simulink model "Experiment_2_cs"  (Simulink 8.4)
settings: Solver=ode5  SolverMode=SingleTasking  StartTime=0.0  StopTime=inf  FixedStep=1/100  RelTol=1e-3
PreLoadFcn:
  | mbxruntime.callbacks.PreLoadFcn(bdroot);
PostLoadFcn:
  | mbxruntime.callbacks.PostLoadFcn(bdroot);
InitFcn:
  | mbxruntime.callbacks.InitFcn(bdroot);
StartFcn:
  | mbxruntime.callbacks.StartFcn(bdroot);
StopFcn:
  | mbxruntime.callbacks.StopFcn(bdroot);
undefined symbols (not defined in the file or in its folder): dfreq, gray, InitImageOutputDir, Rec, SDTV, strel, warningInitialVelocity, x0
libraries: simulink x43, PreScanSimulinkLibrary x19, visiontextngfix x15, simulink_extras x11, visionconversions x3, PreScanUsefulBlocks x3, visionsinks x2, visionstatistics x1, visionmorphops x1, visionanalysis x1
(part 8 of 8)

== matlab function Audi_A8_1/ENABLED/PPS Model/Pedestrian detection/Blob Analysis/PEDES1 ==
  data: inpoints output double; pts input double
function inpoints= points(pts)
%#eml
inpoints = pts;
inpoints(1, :)=pts(2, :);
inpoints(2, :)=pts(1, :);

for i = 1 : size(inpoints, 2)
    if inpoints(1, i) ~= -1
        inpoints(1, i)=inpoints(1, i) +1;
    end
    if inpoints(2, i) ~= -1
        inpoints(2, i)=inpoints(2, i) +1;
    end
end

== matlab function Audi_A8_1/ENABLED/V2X_210_Generic_Expander/Expander ==
  data: u input Bus: PRESCAN_V2X_USER_GENERIC_MESSAGE; y output Bus: PRESCAN_V2X_FIXED_GENERIC_MESSAGE; z input Bus: PRESCAN_V2X_FIXED_GENERIC_MESSAGE
function y = fcn(u, z)
%#eml

y = V2X_GENERIC_expander(u, z);

== matlab function Audi_A8_1/ENABLED/PathFollower_Preview_1/LateralController/Calculate delta steering error/eml_delta_steering_error ==
  data: v_x_vehicle input double; v_x_vehicle_Min input double; t_Preview_LatCtrl input double; delta_steeringwheeltotal output double; v_y_vehicle input double; yawrate_vehicle input double; CorneringStiffness_Tyres_Front input double; CorneringStiffness_Tyres_Rear input double; m_vehicle_total input double; inertia_z_vehicle_total input double; e_Lat input double size=10; Pos_x_CoG_Vehicle input double; wheelbase input double; RefreshCounter parameter double
function delta_steeringwheeltotal = eml_delta_steering_error(v_x_vehicle,v_x_vehicle_Min,t_Preview_LatCtrl,v_y_vehicle,yawrate_vehicle,CorneringStiffness_Tyres_Front,CorneringStiffness_Tyres_Rear,m_vehicle_total,inertia_z_vehicle_total,e_Lat,Pos_x_CoG_Vehicle,wheelbase,RefreshCounter)

delta_steeringwheeltotal = emlfcn_delta_steering_error(v_x_vehicle,v_x_vehicle_Min,t_Preview_LatCtrl,v_y_vehicle,yawrate_vehicle,CorneringStiffness_Tyres_Front,CorneringStiffness_Tyres_Rear,m_vehicle_total,inertia_z_vehicle_total,e_Lat,Pos_x_CoG_Vehicle,wheelbase,RefreshCounter);

% end function

== matlab function Audi_A8_1/ENABLED/PPS Model/Pedestrian detection/PEDES3 ==
  data: inpoints output double; pts input double
function inpoints= points(pts)
%#eml
inpoints = pts;
inpoints(1, :)=pts(2, :);
inpoints(2, :)=pts(1, :);
inpoints(3, :)=pts(4, :);
inpoints(4, :)=pts(3, :);

for i = 1 : size(inpoints, 2)
    if inpoints(1, i) ~= -1
        inpoints(1, i)=inpoints(1, i) +1;
    end
    if inpoints(2, i) ~= -1
        inpoints(2, i)=inpoints(2, i) +1;
    end
end

== matlab function Audi_A8_1/ENABLED/PPS Model/Pedestrian detection/PEDES10 ==
  data: inpoints output double; pts input double
function inpoints= points(pts)
%#eml
inpoints = pts;
inpoints(1, :)=pts(2, :);
inpoints(2, :)=pts(1, :);

for i = 1 : size(inpoints, 2)
    if inpoints(1, i) ~= -1
        inpoints(1, i)=inpoints(1, i) +1;
    end
    if inpoints(2, i) ~= -1
        inpoints(2, i)=inpoints(2, i) +1;
    end
end

== matlab function Audi_A8_1/ENABLED/PPS Model/Pedestrian detection/Blob Analysis/PEDES4 ==
  data: inpoints output double; pts input double
function inpoints= points(pts)
%#eml
inpoints = pts;
inpoints(1, :)=pts(2, :);
inpoints(2, :)=pts(1, :);
inpoints(3, :)=pts(4, :);
inpoints(4, :)=pts(3, :);

for i = 1 : size(inpoints, 2)
    if inpoints(1, i) ~= -1
        inpoints(1, i)=inpoints(1, i) +1;
    end
    if inpoints(2, i) ~= -1
        inpoints(2, i)=inpoints(2, i) +1;
    end
end

== matlab function Audi_A8_1/ENABLED/PPS Model/Pedestrian detection/PEDES4 ==
  data: inpoints output double; pts input double
function inpoints= points(pts)
%#eml
inpoints = pts;
for i=1:size(pts,1)
    for j=1:2
         inpoints(i,j)=pts(i,j)+1;
    end
     for j=3:4
         inpoints(i,j)=pts(i,j)-1;
    end
end

== matlab function Audi_A8_1/ENABLED/PPS Model/Pedestrian detection/Blob Analysis/MATLAB Function ==
  data: u input double; y output double
function y = fcn(u)
%#codegen

y = u(1:2, :);

== matlab function Audi_A8_1/ENABLED/PPS Model/Pedestrian detection/PEDES6 ==
  data: inpoints output double; pts input double
function inpoints= points(pts)
%#eml
inpoints = pts;
inpoints(1, :)=pts(2, :);
inpoints(2, :)=pts(1, :);

for i = 1 : size(inpoints, 2)
    if inpoints(1, i) ~= -1
        inpoints(1, i)=inpoints(1, i) +1;
    end
    if inpoints(2, i) ~= -1
        inpoints(2, i)=inpoints(2, i) +1;
    end
end

== matlab function Audi_A8_1/ENABLED/PPS Model/Pedestrian detection/PEDES8 ==
  data: inpoints output double; pts input double
function inpoints= points(pts)
%#eml
inpoints = pts;
inpoints(1, :)=pts(2, :);
inpoints(2, :)=pts(1, :);

for i = 1 : size(inpoints, 2)
    if inpoints(1, i) ~= -1
        inpoints(1, i)=inpoints(1, i) +1;
    end
    if inpoints(2, i) ~= -1
        inpoints(2, i)=inpoints(2, i) +1;
    end
end

== matlab function Audi_A8_1/ENABLED/PPS Model/Pedestrian detection/Blob Analysis/PEDES3 ==
  data: inpoints output double; pts input double
function inpoints= points(pts)
%#eml
inpoints = pts;
inpoints(1, :)=pts(2, :);
inpoints(2, :)=pts(1, :);
for i = 1 : size(inpoints, 2)
    if inpoints(1, i) ~= -1
        inpoints(1, i)=inpoints(1, i) -1;
    end
    if inpoints(2, i) ~= -1
        inpoints(2, i)=inpoints(2, i) -1;
    end
end

== matlab function Audi_A8_1/ENABLED/PPS Model/Pedestrian detection/Blob Analysis/Embedded MATLAB Function1 ==
  data: centroid input double; centout output double; bbox input double; bboxout output double; majoraxis input double; minoraxis input double; orientation input double; eccentricity input double; label input double; label_out output double size=[400 550]; im_x input double; im_y input double; posObj_subim input double; liminf_x input double; liminf_y input double; posObj_im output double
function [centout,bboxout,label_out,posObj_im] = select_blobs(centroid,bbox,majoraxis,minoraxis,orientation,eccentricity,label,im_x,im_y,posObj_subim, liminf_x,liminf_y)
%#eml
a=1;
centroid=int32(centroid);
centout=int32(zeros(2,size(centroid,2)));
bboxout=int32(zeros(4,size(bbox,2)));
label_out=zeros(size(label,1),size(label,2));
posObj_im=posObj_subim;
for i=1:size(posObj_subim,2)
    posObj_im(:,i)=posObj_subim(:,i)+[liminf_y;liminf_x];
end

for i=1:size(orientation,2)
    touch=0;
    if orientation(1,i)>=180
         or_val=360-orientation(1,i);
     else
         or_val=orientation(1,i);
     end
     lr=bbox(1,i)+1;
     lh=lr+bbox(3,i)-1;
     lc=bbox(2,i)+1;
     lw=lc+bbox(4,i)-1;
      if (bbox(1,i)==0)
          touch=touch+1;
      end
      if (bbox(2,i)==0)
          touch=touch+1;
      end
      if(im_y-centroid(1,i)-(bbox(4,i)/2)<2)
          touch=touch+1;
      end
      if (im_x-centroid(2,i)-(bbox(3,i)/2)<2)
          touch=touch+1;
      end
     
     if (abs(or_val)>55)&&(abs(or_val)<145)&&((majoraxis(i)/minoraxis(i))>1.5)&&((majoraxis(i)/minoraxis(i))<3)&&(eccentricity(i)>0)&&(eccentricity(i)<1)&&(touch<2)
         bboxout(1:2,a)= bbox(1:2,i)+int32([liminf_y;liminf_x]);
         bboxout(3:4,a)= bbox(3:4,i);
         centout(:,a)= centroid(:,i)+int32([liminf_y;liminf_x]);
         label_out(lr:lh,lc:lw)=a;
         a=a+1;
     else
        label_out(lr:lh,lc:lw)=0;
     end
end

== matlab function Audi_A8_1/ENABLED/PPS Model/Pedestrian detection/PEDES7 ==
  data: inpoints output double; pts input double
function inpoints= points(pts)
%#eml
inpoints = pts;
inpoints(1, :)=pts(2, :);
inpoints(2, :)=pts(1, :);
inpoints(3, :)=pts(4, :);
inpoints(4, :)=pts(3, :);

for i = 1 : size(inpoints, 2)
    if inpoints(1, i) ~= -1
        inpoints(1, i)=inpoints(1, i) +1;
    end
    if inpoints(2, i) ~= -1
        inpoints(2, i)=inpoints(2, i) +1;
    end
end

== matlab function Audi_A8_1/ENABLED/PPS Model/Pedestrian detection/Blob Analysis/Embedded MATLAB Function2 ==
  data: nbboxout input double; label input double; r_label output double; color output double
function [r_label,color] = r_labels(nbboxout,label)
%#eml
n=size(nbboxout,2);
r_label=zeros(1,n);
color=zeros(1,n);
not_before=1;
a=1;
for i=1:size(label,1)
    for j=1:size(label,2)
        if (a==1)
            if (label(i,j)~=0)
                r_label(1,a)=label(i,j);
                a=a+1;
            end
        else
             if (label(i,j)~=0)
                 for h=1:a
                     if(label(i,j)~=r_label(1,h))
                         not_before=1;
                     else
                         not_before=0;
                         break
                     end
                 end
                 if not_before==1
                     r_label(1,a)=label(i,j);
                     a=a+1;
                 end
             end
        end 
    end 
end
color(1,:)=2;

== matlab function Audi_A8_1/ENABLED/PPS Model/Pedestrian detection/PEDES9 ==
  data: inpoints output double; pts input double
function inpoints= points(pts)
%#eml
inpoints = pts;
for i=0:(size(pts,1)/2-1)    
    inpoints(2*i+1)=pts(2*i+2);
    inpoints(2*i+2)=pts(2*i+1);
end

== matlab function Audi_A8_1/ENABLED/PPS Model/Pedestrian detection/POSITION ==
  data: flag input double size=TISdet; theta input double size=TISdet; posit output double; range input double; xs_m output double; ys_m output double; TISdet parameter double; TISMaxRange parameter double
function [posit,xs_m,ys_m]= positt(flag,theta,range,TISdet, TISMaxRange)
%#codegen
xposit = zeros(1,TISdet);
yposit = zeros(1,TISdet);
posit = zeros(2,TISdet);
xs_m = zeros(1,TISdet);
ys_m = zeros(1,TISdet);
X_offset = 3.9 - 1.9;                                   %Offset Between Camera and Radar Positions
Z_offset = 0.42 - 1.28;                                 %Offset Between Camera and Radar Positions

f = 0.0075;                                             %Focal Length
sx = 0.0048;                                            %Pixel Width
%Maximum Camera Cooridnates%
u_max = TISMaxRange * sin(23.1*pi/180);                          %radar range = 40m, camera fov = 46.2 degrees 
v_max = TISMaxRange * cos(23.1*pi/180);

for i=1:TISdet
    if (flag(i)==0) || (theta(i)==0)
        xposit(i) = 0;
        posit(1,i) = 0;
    elseif (flag(i)~=0)
        theta_aux = -theta(i);      
        
        X = range(i)*cos(theta_aux*pi/180);
        Y = range(i)*sin(theta_aux*pi/180);
        
        xs_m(i) = Y;        
        ys_m(i) = X;
        %Camera 3-D Coordinates%
        X_c = X + X_offset;
        Y_c = Y;

        %Camera Pixel Coordinates%
        u_r_new = (Y*f*500)/(sx*u_max);
      
        %Conversion of xc to pixel value%
        xposit(i)= 250 + u_r_new;
        yposit(i)=188;
    end
     posit(2,i)=round(xposit(i));
     posit(1,i)=round(yposit(i));
end

== matlab function Audi_A8_1/ENABLED/PPS Model/Pedestrian detection/Image processing/Embedded MATLAB Function ==
  data: im output double size=[375 500]; image input double
function im = sub_image(image)
%#eml
im=zeros(size(image,1),size(image,2));
for i=1:size(image,1)
    for j=1:size(image,2)
        if (image(i,j)==0)
            im(i,j)=1;
        else
            im(i,j)=0;
        end
    end
end

== matlab function Audi_A8_1/ENABLED/PPS Model/Pedestrian detection/PEDES ==
  data: CentAlarms output double; PosObj_subim input double; Centroid_subim input double; alarms output double size=TISdet; BBox input double; BBox_det output double; TISdet parameter double
function [CentAlarms,alarms,BBox_det]= pedes(PosObj_subim, Centroid_subim,BBox,TISdet)
%#eml
CentAlarms=int32(zeros(2,size(PosObj_subim,2)));
alarms=zeros(size(PosObj_subim,2),1);
BBox_det=int32(zeros(4,size(BBox,2)));
a=1;
for i=1:size(PosObj_subim,2)
    for j=1:size(Centroid_subim,2)
        if (Centroid_subim(1,j)~=0)||(Centroid_subim(2,j)~=0)
            if (abs(Centroid_subim(2,j)-PosObj_subim(2,i))<15)||(abs(Centroid_subim(1,j)-PosObj_subim(1,i))<15)%(PosObj_subim(1,i))>BBox(1,j)&&(PosObj_subim(1,i))<(BBox(1,j)+BBox(3,j))
                alarms(a,1)=1;
                CentAlarms(:,a)=PosObj_subim(:,i);%Centroid_subim(:,j);
                BBox_det(:,a)=BBox(:,i);
            end
        end
    end
    a=a+1;
end

== matlab function Audi_A8_1/ENABLED/PPS Model/Pedestrian detection/PEDES1 ==
  data: Im input double size=[375 500]; Imout output double size=[375 500 3]
function Imout = imag(Im)
%#eml
Imout=128*ones(size(Im,1),size(Im,2),3);
Imout(:,:,1)=Im;

== matlab function Audi_A8_1/ENABLED/PPS Model/Pedestrian detection/PEDES2 ==
  data: Im input double size=[375 500]; Imout output double size=[375 500 3]
function Imout = imag(Im)
%#eml
Imout=128*ones(size(Im,1),size(Im,2),3);
Imout(:,:,1)=Im;

== matlab function Audi_A8_1/ENABLED/PPS Model/Pedestrian detection/scaling_crop ==
  data: im input double; PosObj input double; X input double; Y input double; sub_im output double size=[375 500]; posObj_subim output double; im_x output double; im_y output double; liminf_x output double; liminf_y output double; rectangle output double
function [sub_im,posObj_subim,im_x,im_y,liminf_x, liminf_y,rectangle]=escaling(im,PosObj,X,Y)

minPx=size(im,2);
minPy=size(im,1);
maxPx=0;
maxPy=0;
detected=0;
mino=0;
maxo=0;
for i=1:size(PosObj,2)
    if PosObj(2,i)~=0
        if(PosObj(2,i)<minPx)
            minPx=PosObj(2,i);
            minPy=PosObj(1,i);
            mino=i;
        end
        if (PosObj(2,i)>maxPx)
            maxPx=PosObj(2,i);
            maxPy=PosObj(1,i);
            maxo=i;
        end
        detected=detected+1;
    end
end
if (detected==0)
    liminf_x=size(im,2);
    limsup_x=size(im,2);
    liminf_y=size(im,1);
    limsup_y=size(im,1);
 
 else
   
  %%For horizontal and vertical position
   
  if (mino~=0) 
    liminf_x= round(minPx-((40-round(1.6*Y(mino)))*2));
    liminf_y= round(minPy-((100-round(4.5*Y(mino)))*2));
    
  else
     liminf_x=1;
     liminf_y=1;
  end
   if (maxo~=0)   
    limsup_x= abs(round(maxPx+((40-round(1.6*Y(maxo)))*2)));
    limsup_y= abs(round(maxPy+((100-round(5*Y(maxo)))*2)));
   else
       limsup_x=size(im,2);
       limsup_y=size(im,1);
   end

end

  if (liminf_x<1)
         liminf_x=1;
  end
    
  if (limsup_x>size(im,2))
        limsup_x=size(im,2);
  end
    
  if (liminf_y<1)
       liminf_y=1;
  end
    
  if (limsup_y>=size(im,1))
       limsup_y=size(im,1);
  end
  
  if (liminf_y > size(im,1))
        liminf_y = size(im,1);
  end
    
   posObj_subim=zeros(2,size(PosObj,2));
   a=1;
    
    for i=1:size(PosObj,2)
        if (PosObj(2,i)~=0)
            posObj_subim(:,a)=[PosObj(1,i)-liminf_y;PosObj(2,i)-liminf_x];
            a=a+1;
        end
    end

sub_im=im(liminf_y:limsup_y,liminf_x:limsup_x);

if length( sub_im ) < 3
    sub_im = zeros(3,3,'uint8');
end


im_x=limsup_x-liminf_x;
im_y=limsup_y-liminf_y;
rectangle=[liminf_y liminf_x im_y im_x];

== matlab function Audi_A8_1/ENABLED/PPS Model/Radar detection/Straight road segment/Relative velocity2/Embedded MATLAB Function1 ==
  data: r input double; yp2 output double; yp1 input double; K1 input double; K2 output double; TISdet parameter double; TISMaxRange parameter double
function [yp2, K2] = modif(r, yp1, K1, TISdet, TISMaxRange)
%#eml
% Interpolating yp value.

K2 = K1;
yp2 = yp1;

d = 50;

% Adding point
for i = 1 : TISdet
   if r(i) ~= 150
      K2(i,1:d-1) = K2(i,2:d);
      K2(i,d) = yp1(i);
   end
end

% Choosing what to take
for i = 1 : TISdet
    s = 0;
    suma = 0;
    for j = 1 : 50
        if K2(i,j) ~= 0
            suma = suma + K2(i,j);
            s = s + 1;
        end
    end
    yp2(i) = suma/s;
end

% Returning, if object is not detected
for i = 1: TISdet
    if r(i) == TISMaxRange && yp1(i) == 0
        K2(i,:,:) = zeros(d,1);
        yp2(i) = 0;
    end    
end

== matlab function Audi_A8_1/ENABLED/PPS Model/Pedestrian detection/PEDES5 ==
  data: blob_subim_proces output double; sub_im input double size=[375 500]; limx_inf input double; limy_inf input double; im_x input double; im_y input double
function blob_subim_proces = blob_subim(sub_im, limx_inf, limy_inf,im_x,im_y)
%#eml
blob_subim_proces=single(zeros(375,500));

limx_sup=limx_inf+im_x;
limy_sup=limy_inf+im_y;

% Assigned the superior and inferior limit 
limx_sup_sorted=max([limx_sup limx_inf]);
limx_inf_sorted=min([limx_sup limx_inf]);
limy_inf_sorted=min([limy_sup limy_inf]);
limy_sup_sorted=max([limy_sup limy_inf]);


[nn, mm] = size( sub_im );
if ( nn <= 3 ) && ( mm <= 3 )
    sub_im = 0;
    % Create a zeros matrix of size (im_y,im_x)
    if im_x~=0 || im_y~=0
        im_x=abs(im_x);
        im_y=abs(im_y);
        assert(im_x<1000);
        assert(im_y<1000);
        sub_im=zeros(im_y+1,im_x+1);
    end
end


blob_subim_proces(limy_inf_sorted:limy_sup_sorted,limx_inf_sorted:limx_sup_sorted)=sub_im;

== matlab function Audi_A8_1/ENABLED/PPS Model/Radar detection/Straight road segment/Relative velocity2/Translation ==
  data: v input double; xpd input double; xp_dot output double; TISdet parameter double
function xp_dot = trans(v, xpd, TISdet)
%#codegen
%Translation of the value

xp_dot = xpd;
for i = 1 : TISdet
    if xpd(i) == v
        xp_dot(i) =0;
    end
end
end

== matlab function Audi_A8_1/ENABLED/PPS Model/Radar detection/Straight road segment/THETA Derivative1/Deriv correction ==
  data: th input double; thp input double; thd input double; th_dot output double; TISdet parameter double
function th_dot = stopping(th, thp, thd, TISdet)
%#codegen
% Stopping if nothing is detected.

th_dot = thd;
for i = 1 : TISdet
    if (th(i)==0 && thp(i)~=0) || (th(i)~=0 && thp(i)==0)
        th_dot(i) = 0;
    end
end
end

== matlab function Audi_A8_1/ENABLED/PPS Model/Radar detection/Straight road segment/THETA Derivative1/Theta extrapolation ==
  data: r input double; th1 input double; th2 output double; thd input double; time input double; K1 input double; K2 output double; TISdet parameter double; TISMaxRange parameter double
function [th2, K2] = modif(r, th1, thd, time, K1, TISdet, TISMaxRange)
%#codegen
% Interpolating theta value.

K2 = K1;
th2 = th1;

d = 10;

% Finding points used in interpolation/extrapolation.
for i = 1 : TISdet
    if thd(i) ~= 0
        K2(i,1:d-1,:) = K2(i,2:d,:);
        K2(i,  d,1) = time;
        K2(i,  d,2) = th1(i);
    end
end

% Extrapolation
for i = 1 : TISdet
    j = 1;
    while j < d+1 && K2(i,j,1) == 0
        j = j + 1;
    end
    
    if j > d-2
        th2(i) = th1(i);
    else
        th2(i) = interp1(K2(i,d-2:d,1),K2(i,d-2:d,2),time,'linear','extrap');
    end
end

% Returning, if object is not detected
for i = 1: TISdet
    if r(i) == TISMaxRange && th1(i) == 0
        K2(i,:,:) = zeros(d,2);
        th2(i) = 0;
    end    
end

end

== matlab function Audi_A8_1/ENABLED/MATLAB Function2 ==
  data: carX input double; pedR output double; carY input double; carZ input double; carRotZ input double; pedX input double; pedY input double; pedZ input double; sensorCorrX input double; sensorCorrY input double; sensorCorrZ input double; pedTheta output double; pedPhi output double
function [pedR,pedTheta,pedPhi] = calculateTISdataFunc(carX,carY,carZ,carRotZ,pedX,pedY,pedZ,sensorCorrX,sensorCorrY,sensorCorrZ)
%#codegen
TcarMat = [1 0 0 carX ; 0 1 0 carY ; 0 0 1 carZ ; 0 0 0 1];

RcarMat = [cosd(carRotZ) -sind(carRotZ) 0 0;
    sind(carRotZ) cosd(carRotZ) 0 0;
    0 0 1 0;
    0 0 0 1];

TsensorMat = [1 0 0 sensorCorrX ; 0 0 1 sensorCorrY ; 0 1 0 sensorCorrZ ; 0 0 0 1];

FcarMat = TcarMat*RcarMat*TsensorMat*[0;0;0;1];

pedR = zeros(length(pedX),1);
pedTheta = zeros(length(pedX),1);
pedPhi = zeros(length(pedX),1);

for i = 1:length(pedX)

[pedThetaTemp,pedPhiTemp,pedRTemp] = cart2sph(pedX(i) - FcarMat(1), pedY(i) - FcarMat(2), pedZ - FcarMat(3));

pedR(i) = pedRTemp;
pedTheta(i) = -(pedThetaTemp*180/pi-carRotZ);
pedPhi(i) = pedPhiTemp*180/pi;

end

== matlab function Audi_A8_1/ENABLED/MATLAB Function ==
  data: pedR_self input double; pedR_Array output double; pedTheta_self input double; dVel_self input double; pedTheta_Array output double; dVel_Array output double; pedR_rcvd input double; pedTheta_rcvd input double; dVel_rcvd input double
function [pedR_Array,pedTheta_Array,dVel_Array] = adaptDataFunc(pedR_self,pedTheta_self,dVel_self,pedR_rcvd,pedTheta_rcvd,dVel_rcvd)

pedR_Array = zeros(32,1);
pedTheta_Array = zeros(32,1);
dVel_Array = zeros(32,1);

for i=1:length(pedR_self)
    pedR_Array(i) = pedR_self(i);
    pedTheta_Array(i) = pedTheta_self(i);
    dVel_Array(i) = dVel_self(i);
end

for i=1:length(pedR_rcvd)
    pedR_Array(i + length(pedR_self)) = pedR_rcvd(i);
    pedTheta_Array(i + length(pedR_self)) = pedTheta_rcvd(i);
    dVel_Array(i + length(pedR_self)) = dVel_rcvd(i);
end

== matlab function BMW_Z3_1/ENABLED/MATLAB Function ==
  data: carX input double; pedResultX output double; carY input double; carZ input double; carRotZ input double; pedR input double; pedTheta input double; pedPhi input double; sensorCorrX input double; sensorCorrY input double; sensorCorrZ input double; pedResultY output double; pedResultZ output double
function [pedResultX,pedResultY,pedResultZ] = calculatePositionFunc(carX,carY,carZ,carRotZ,pedR,pedTheta,pedPhi,sensorCorrX,sensorCorrY,sensorCorrZ)

TcarMat = [1 0 0 carX ; 0 1 0 carY ; 0 0 1 carZ ; 0 0 0 1];
TsensorMat = [1 0 0 sensorCorrX ; 0 1 0 sensorCorrY ; 0 0 1 sensorCorrZ ; 0 0 0 1];
RcarMat = [cosd(carRotZ) -sind(carRotZ) 0 0 ;
        sind(carRotZ) cosd(carRotZ) 0 0;
        0 0 1 0;
        0 0 0 1];
    
pedResultX = zeros(length(pedR),1);
pedResultY = zeros(length(pedR),1);
pedResultZ = zeros(length(pedR),1);

for i = 1:length(pedR)
    
    [xPed,yPed,zPed] = sph2cart(-pedTheta(i)*pi/180,pedPhi*pi/180,pedR(i));
    
    TpedMat = [1 0 0 xPed ; 0 1 0 yPed ; 0 0 1 zPed ; 0 0 0 1];

    ResultMat = TcarMat*RcarMat*TsensorMat*TpedMat*[0;0;0;1];

    pedResultX(i) = ResultMat(1);
    pedResultY(i) = ResultMat(2);
    pedResultZ(i) = ResultMat(3);

end

== matlab function Audi_A8_1/ENABLED/MATLAB Function1 ==
  data: carX input double; dopplerVelocity output double; carY input double; carZ input double; carAngle input double; carVelocity input double; pedX input double; pedY input double; pedZ input double; dTranslationX input double; dTranslationY input double; dTranslationZ input double; sensorX input double; sensorY input double; sensorZ input double
function dopplerVelocity = relativeVelocity(carX,carY,carZ,carAngle,carVelocity,pedX,pedY,pedZ,dTranslationX,dTranslationY,dTranslationZ,sensorX,sensorY,sensorZ)

rotMat = [cosd(carAngle) -sind(carAngle);
    sind(carAngle) cosd(carAngle)];

sensorMat = rotMat*[sensorX ; sensorY];

carVelX = carVelocity*cosd(carAngle);
carVelY = carVelocity*sind(carAngle);

carVelMat = rotMat\[carVelX ; carVelY];

carMat = [carX + sensorMat(1) ; carY + sensorMat(2)];

dopplerVelocity = zeros(length(pedX),1);

for i = 1:length(pedX)
   
    Vcp = [pedX(i) - carMat(1) ; pedY(i) - carMat(2)];

    Vdv = rotMat\[dTranslationX(i) ; dTranslationY(i)];
    
    Vdv = Vdv - carVelMat;
    
    Vcp = rotMat\Vcp;
    
    dopplerVelocity(i) = dot(Vdv,Vcp)/norm(Vcp);
    
end

== matlab function BMW_Z3_1/ENABLED/MATLAB Function3 ==
  data: carAngle input double; carVelocity input double; dTranslationX output double; dopplerTX input double; dopplerTY input double; dTranslationY output double
function [dTranslationX,dTranslationY] = globalAxisConversion(carAngle,carVelocity,dopplerTX,dopplerTY)

rotMat = [cosd(carAngle) -sind(carAngle);
    sind(carAngle) cosd(carAngle)];

carVelX = carVelocity*cosd(carAngle);
carVelY = carVelocity*sind(carAngle);

carVelMat = [carVelX ; carVelY];

dTranslationX = zeros(length(dopplerTX),1);
dTranslationY = zeros(length(dopplerTY),1);

for i = 1:length(dopplerTX)
    
    Vdv = rotMat*[dopplerTX(i);dopplerTY(i)];
    
    Vdv = Vdv + carVelMat;
    
    dTranslationX(i) = Vdv(1);
    dTranslationY(i) = Vdv(2);

end
